simulink model "lect10_slides_ex1"  (R2023b)
settings: Solver=VariableStepAuto  StartTime=0.0  StopTime=25  RelTol=1e-3
values from neighbouring files (symbols this model uses):
  A = [0   1 ... (first row only)    [lect10_slides_ex1.m]    (also in untitled.m = [-8.8487 + (a-b)/5,     -0.0399,              -5.55 + (c+d)/)
  B = [1 0 ... (first row only)    [lect10_slides_ex1.m]    (also in untitled.m = [0.0564+(b)/(10+c),           0.0319)
  C = [1 0.5 ... (first row only)    [lect10_slides_ex1.m]    (also in untitled.m = [-3.2988,           -2.1932+(10*c+d)/(100+5*a), 0.0370,  -0.)
  F = inv(B_star)    [lect10_slides_ex1.m]
  K = inv(B_star) * C_star_star    [lect10_slides_ex1.m]
  x_0 = [0.5; -0.1; 0.3; -0.8;]    [untitled.m]
settings Model: Creator=john  LastModifiedBy=john

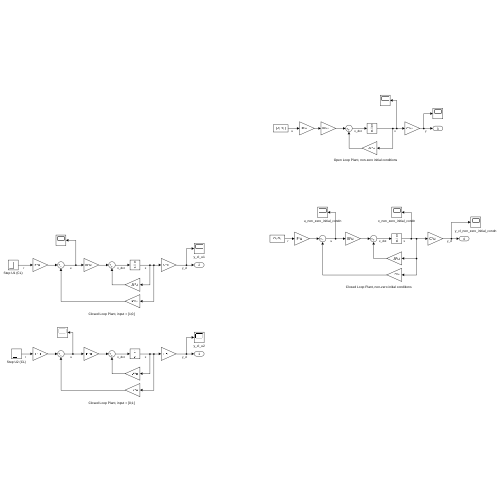
[thumbnail: Simulink's stored preview of the top-level diagram]
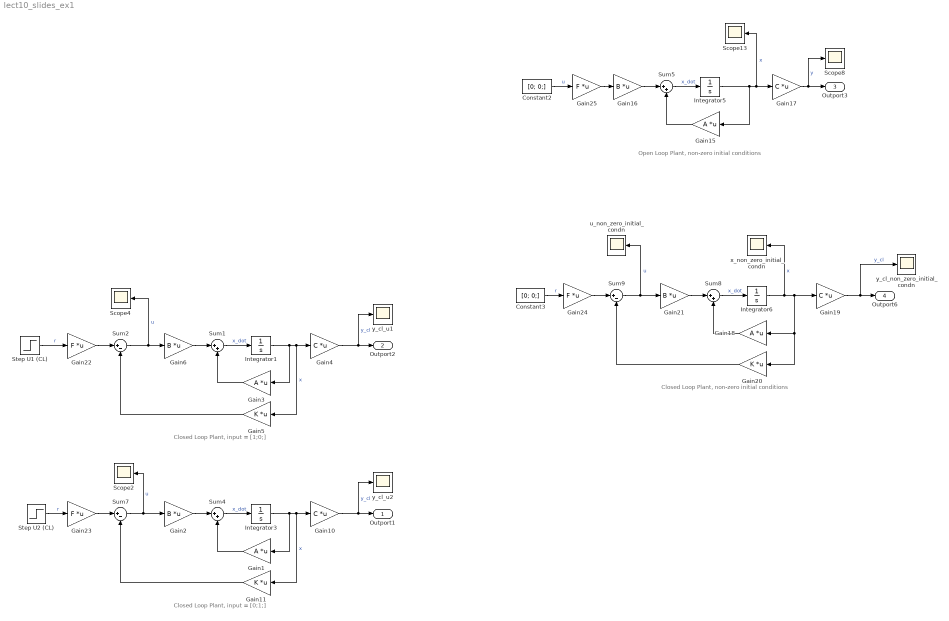
== system lect10_slides_ex1 ==
  note: Closed Loop Plant, input = [0;1;]
  note: Closed Loop Plant, input = [1;0;]
  note: Open Loop Plant, non-zero initial conditions
  note: Closed Loop Plant, non-zero initial conditions
  Constant2 : Constant  Value=[0; 0;]
  Constant3 : Constant  Value=[0; 0;]
  Gain{1,3,15,18} (4 alike) : Gain  Gain=A  Multiplication=Matrix(K*u)
  Gain{4,10,17,19} (4 alike) : Gain  Gain=C  Multiplication=Matrix(K*u)
  Gain11 : Gain  Gain=K  Multiplication=Matrix(K*u)
  Gain{2,6,16,21} (4 alike) : Gain  Gain=B  Multiplication=Matrix(K*u)
  Gain20 : Gain  Gain=K  Multiplication=Matrix(K*u)
  Gain{22..25} (4 alike) : Gain  Gain=F  Multiplication=Matrix(K*u)
  Gain5 : Gain  Gain=K  Multiplication=Matrix(K*u)
  Integrator1 : Integrator
  Integrator3 : Integrator
  Integrator5 : Integrator  InitialCondition=x_0
  Integrator6 : Integrator  InitialCondition=x_0
  Scope{2,4,8,13} (4 alike) : Scope
  Step U1 (CL) : Step  Time=0  Before=[0; 0;];  After=[1; 0;];  SampleTime=0
  Step U2 (CL) : Step  Time=0  Before=[0; 0;];  After=[0; 1;];  SampleTime=0
  Sum{1,4..5,8} (4 alike) : Sum  Inputs=|++
  Sum2 : Sum  Inputs=|+-
  Sum7 : Sum  Inputs=|+-
  Sum9 : Sum  Inputs=|+-
  u_non_zero_initial_condn : Scope
  x_non_zero_initial_condn : Scope
  y_cl_non_zero_initial_condn : Scope
  y_cl_u1 : Scope
  y_cl_u2 : Scope
  Outport1 : Outport
  Outport2 : Outport  Port=2
  Outport3 : Outport  Port=3
  Outport6 : Outport  Port=4
  wires:
  Gain10/1 -> y_cl_u2/1, Outport1/1  "y_cl"
  Integrator3/1 -> Gain1/1, Gain11/1, Gain10/1  "x"
  Gain1/1 -> Sum4/2
  Gain11/1 -> Sum7/2
  Sum4/1 -> Integrator3/1  "x_dot"
  Sum7/1 -> Scope2/1, Gain2/1  "u"
  Step U2 (CL)/1 -> Gain23/1  "r"
  Gain2/1 -> Sum4/1
  Gain4/1 -> y_cl_u1/1, Outport2/1  "y_cl"
  Gain6/1 -> Sum1/1
  Sum1/1 -> Integrator1/1  "x_dot"
  Integrator1/1 -> Gain3/1, Gain5/1, Gain4/1  "x"
  Gain5/1 -> Sum2/2
  Sum2/1 -> Scope4/1, Gain6/1  "u"
  Step U1 (CL)/1 -> Gain22/1  "r"
  Gain3/1 -> Sum1/2
  Sum5/1 -> Integrator5/1  "x_dot"
  Integrator5/1 -> Gain17/1, Scope13/1, Gain15/1  "x"
  Gain17/1 -> Scope8/1, Outport3/1  "y"
  Gain16/1 -> Sum5/1
  Gain15/1 -> Sum5/2
  Gain21/1 -> Sum8/1
  Gain20/1 -> Sum9/2
  Sum8/1 -> Integrator6/1  "x_dot"
  Integrator6/1 -> Gain20/1, Gain18/1, Gain19/1, x_non_zero_initial_condn/1  "x"
  Gain19/1 -> y_cl_non_zero_initial_condn/1, Outport6/1  "y_cl"
  Sum9/1 -> u_non_zero_initial_condn/1, Gain21/1  "u"
  Gain18/1 -> Sum8/2
  Constant2/1 -> Gain25/1  "u"
  Constant3/1 -> Gain24/1  "r"
  Gain22/1 -> Sum2/1
  Gain23/1 -> Sum7/1
  Gain24/1 -> Sum9/1
  Gain25/1 -> Gain16/1
